simulink model "Colorspace_Conversion_fixed"  (R2016a)
settings: Solver=VariableStepAuto  StartTime=0.0  StopTime=1  RelTol=1e-3
undefined symbols (not defined in the file): gray
libraries: ModelComposer x27, dspvision x1
settings Model: Creator=ukumar  LastModifiedBy=wesleyl
settings DebuggingCC: InheritedTsInSrcMsg=none

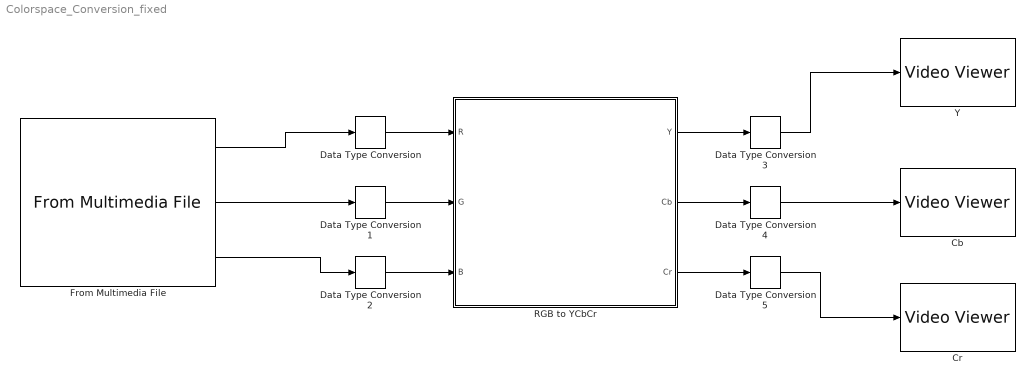
== system Colorspace_Conversion_fixed ==
  "Cb " : VideoViewer  colormapValue=gray(256)  FigPos=[523.4 526 487.2 356]
  "Cr " : VideoViewer  colormapValue=gray(256)  FigPos=[1036.2 531.6 464.8 360]
  Data Type Conversion : ModelComposer/Data Type Conversion  OutDataType=fixed  TypeExp=''  Signedness=Unsigned  WordLength=8  FractionalLength=7  RoundingMode=Truncation to minus infinity  OverflowMode=Wrap around
  Data Type Conversion1 : ModelComposer/Data Type Conversion  OutDataType=fixed  TypeExp=''  Signedness=Unsigned  WordLength=8  FractionalLength=7  RoundingMode=Truncation to minus infinity  OverflowMode=Wrap around
  Data Type Conversion2 : ModelComposer/Data Type Conversion  OutDataType=fixed  TypeExp=''  Signedness=Unsigned  WordLength=8  FractionalLength=7  RoundingMode=Truncation to minus infinity  OverflowMode=Wrap around
  Data Type Conversion3 : ModelComposer/Data Type Conversion  OutDataType=single  TypeExp=''  Signedness=Signed  WordLength=16  FractionalLength=10  RoundingMode=Truncation to minus infinity  OverflowMode=Wrap around
  Data Type Conversion4 : ModelComposer/Data Type Conversion  OutDataType=single  TypeExp=''  Signedness=Signed  WordLength=16  FractionalLength=10  RoundingMode=Truncation to minus infinity  OverflowMode=Wrap around
  Data Type Conversion5 : ModelComposer/Data Type Conversion  OutDataType=single  TypeExp=''  Signedness=Signed  WordLength=16  FractionalLength=10  RoundingMode=Truncation to minus infinity  OverflowMode=Wrap around
  From Multimedia File : dspvision/From Multimedia File  inputFilename=visionface.avi  loop=on  numPlays=inf  outputStreams=Video only  videoDataType=single  audioDataType=int16  inheritSampleTime=on  userDefinedSampleTime=1/30  noAudioOutput=off  isIntensityVideo=off  fourcc=RGB  colorVideoFormat=Separate color signals  outputEOF=off  dataOrg=Column-major  audioFrameSize=1024  computeAudioFrameSize=off  outSamplingMode=Sample based
  RGB to YCbCr : Subsystem
  Y : VideoViewer  colormapValue=gray(256)  FigPos=[32.2 527.6 464 357.6]
  wires:
  From Multimedia File/2 -> Data Type Conversion1/1
  From Multimedia File/3 -> Data Type Conversion2/1
  RGB to YCbCr/1(Y) -> Data Type Conversion3/1
  RGB to YCbCr/2(Cb) -> Data Type Conversion4/1
  RGB to YCbCr/3(Cr) -> Data Type Conversion5/1
  From Multimedia File/1 -> Data Type Conversion/1
  Data Type Conversion/1 -> RGB to YCbCr/1(R)
  Data Type Conversion1/1 -> RGB to YCbCr/2(G)
  Data Type Conversion2/1 -> RGB to YCbCr/3(B)
  Data Type Conversion4/1 -> "Cb "/1
  Data Type Conversion5/1 -> "Cr "/1
  Data Type Conversion3/1 -> Y/1

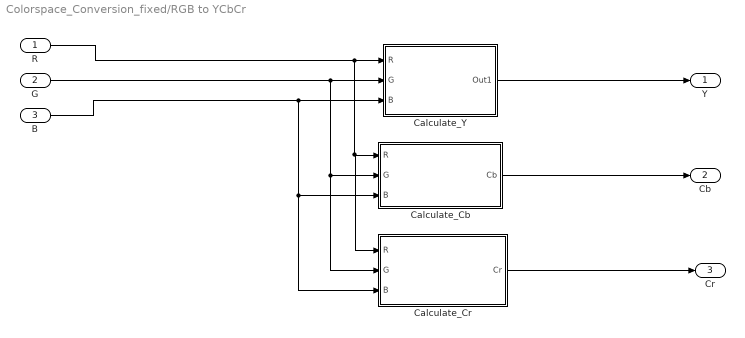
== system Colorspace_Conversion_fixed/RGB to YCbCr ==
  R : Inport
  G : Inport  Port=2
  B : Inport  Port=3
  "Calculate_Cb " : Subsystem
  Calculate_Cr : Subsystem
  "Calculate_Y " : Subsystem
  Y : Outport
  Cb : Outport  Port=2
  Cr : Outport  Port=3
  wires:
  "Calculate_Y "/1(Out1) -> Y/1
  "Calculate_Cb "/1("Cb ") -> Cb/1
  Calculate_Cr/1(Cr) -> Cr/1
  R/1 -> Calculate_Cr/1("R "), "Calculate_Cb "/1("R "), "Calculate_Y "/1("R ")
  G/1 -> Calculate_Cr/2("G "), "Calculate_Cb "/2("G "), "Calculate_Y "/2("G ")
  B/1 -> Calculate_Cr/3(B), "Calculate_Cb "/3(B), "Calculate_Y "/3("B ")

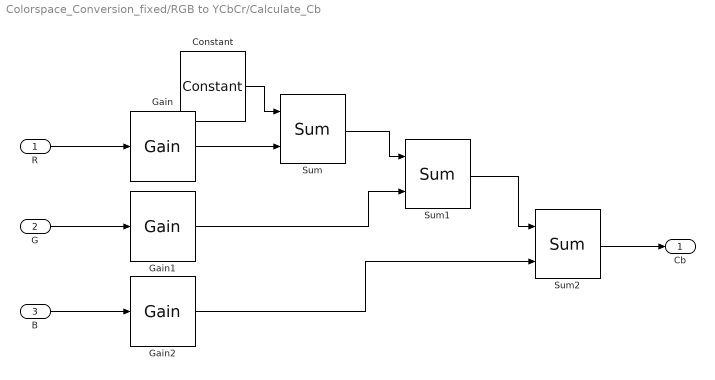
== system Colorspace_Conversion_fixed/RGB to YCbCr/Calculate_Cb  ==
  "R " : Inport
  "G " : Inport  Port=2
  B : Inport  Port=3
  Constant : ModelComposer/Constant  Description=Performs multiplication  Value=128/255  SampleTime=-1  OutDataType=fixed  TypeExp=''  Signedness=Signed  WordLength=8  FractionalLength=7  RoundingMode=Truncation to minus infinity  OverflowMode=Wrap around
  Gain : ModelComposer/Gain  Description=Performs multiplication  Gain=-37.945/256  OutDataType=fixed  TypeExp=''  Signedness=Signed  WordLength=8  FractionalLength=7  RoundingMode=Truncation to minus infinity  OverflowMode=Wrap around  OutputTypeAsInput=off
  Gain1 : ModelComposer/Gain  Description=Performs multiplication  Gain=-74.494/256  OutDataType=fixed  TypeExp=''  Signedness=Signed  WordLength=8  FractionalLength=7  RoundingMode=Truncation to minus infinity  OverflowMode=Wrap around  OutputTypeAsInput=off
  Gain2 : ModelComposer/Gain  Description=Performs multiplication  Gain=112.439/256  OutDataType=fixed  TypeExp=''  Signedness=Signed  WordLength=8  FractionalLength=7  RoundingMode=Truncation to minus infinity  OverflowMode=Wrap around  OutputTypeAsInput=off
  Sum : ModelComposer/Sum
  Sum1 : ModelComposer/Sum
  Sum2 : ModelComposer/Sum
  "Cb " : Outport
  wires:
  Sum2/1 -> "Cb "/1
  "R "/1 -> Gain/1
  "G "/1 -> Gain1/1
  B/1 -> Gain2/1
  Constant/1 -> Sum/1
  Gain/1 -> Sum/2
  Sum/1 -> Sum1/1
  Gain1/1 -> Sum1/2
  Sum1/1 -> Sum2/1
  Gain2/1 -> Sum2/2

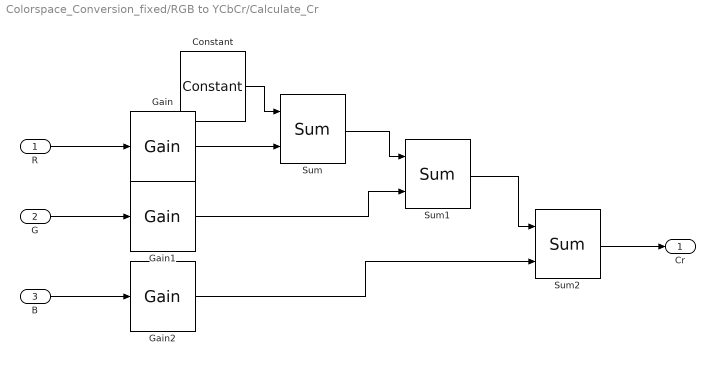
== system Colorspace_Conversion_fixed/RGB to YCbCr/Calculate_Cr ==
  "R " : Inport
  "G " : Inport  Port=2
  B : Inport  Port=3
  Constant : ModelComposer/Constant  Description=Performs multiplication  Value=128/255  SampleTime=-1  OutDataType=fixed  TypeExp=''  Signedness=Signed  WordLength=8  FractionalLength=7  RoundingMode=Truncation to minus infinity  OverflowMode=Wrap around
  Gain : ModelComposer/Gain  Description=Performs multiplication  Gain=112.439/256  OutDataType=fixed  TypeExp=''  Signedness=Signed  WordLength=8  FractionalLength=7  RoundingMode=Truncation to minus infinity  OverflowMode=Wrap around  OutputTypeAsInput=off
  Gain1 : ModelComposer/Gain  Description=Performs multiplication  Gain=-94.154/256  OutDataType=fixed  TypeExp=''  Signedness=Signed  WordLength=8  FractionalLength=7  RoundingMode=Truncation to minus infinity  OverflowMode=Wrap around  OutputTypeAsInput=off
  Gain2 : ModelComposer/Gain  Description=Performs multiplication  Gain=-18.285/256  OutDataType=fixed  TypeExp=''  Signedness=Signed  WordLength=8  FractionalLength=7  RoundingMode=Truncation to minus infinity  OverflowMode=Wrap around  OutputTypeAsInput=off
  Sum : ModelComposer/Sum
  Sum1 : ModelComposer/Sum
  Sum2 : ModelComposer/Sum
  Cr : Outport
  wires:
  Gain2/1 -> Sum2/2
  Sum1/1 -> Sum2/1
  Gain1/1 -> Sum1/2
  Sum/1 -> Sum1/1
  Gain/1 -> Sum/2
  Constant/1 -> Sum/1
  B/1 -> Gain2/1
  "G "/1 -> Gain1/1
  "R "/1 -> Gain/1
  Sum2/1 -> Cr/1

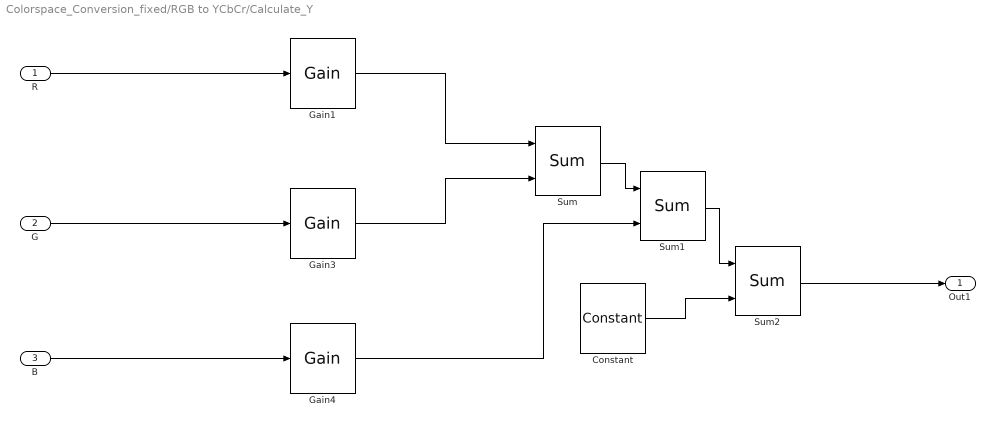
== system Colorspace_Conversion_fixed/RGB to YCbCr/Calculate_Y  ==
  "R " : Inport
  "G " : Inport  Port=2
  "B " : Inport  Port=3
  Constant : ModelComposer/Constant  Description=Performs multiplication  Value=16/255  SampleTime=-1  OutDataType=fixed  TypeExp=''  Signedness=Signed  WordLength=8  FractionalLength=7  RoundingMode=Truncation to minus infinity  OverflowMode=Wrap around
  Gain1 : ModelComposer/Gain  Description=Performs multiplication  Gain=65.738/256  OutDataType=fixed  TypeExp=''  Signedness=Signed  WordLength=8  FractionalLength=7  RoundingMode=Truncation to minus infinity  OverflowMode=Wrap around  OutputTypeAsInput=off
  Gain3 : ModelComposer/Gain  Description=Performs multiplication  Gain=129.057/256  OutDataType=fixed  TypeExp=''  Signedness=Signed  WordLength=8  FractionalLength=7  RoundingMode=Truncation to minus infinity  OverflowMode=Wrap around  OutputTypeAsInput=off
  Gain4 : ModelComposer/Gain  Description=Performs multiplication  Gain=25.064/256  OutDataType=fixed  TypeExp=''  Signedness=Signed  WordLength=8  FractionalLength=7  RoundingMode=Truncation to minus infinity  OverflowMode=Wrap around  OutputTypeAsInput=off
  Sum : ModelComposer/Sum
  Sum1 : ModelComposer/Sum
  Sum2 : ModelComposer/Sum
  Out1 : Outport
  wires:
  Sum/1 -> Sum1/1
  "R "/1 -> Gain1/1
  "B "/1 -> Gain4/1
  "G "/1 -> Gain3/1
  Gain1/1 -> Sum/1
  Gain3/1 -> Sum/2
  Gain4/1 -> Sum1/2
  Sum1/1 -> Sum2/1
  Constant/1 -> Sum2/2
  Sum2/1 -> Out1/1
